simulink model "emldemo_bus_struct"  (Simulink 7.6)
settings: Solver=FixedStepDiscrete  StartTime=0.0  StopTime=1  FixedStep=1  RelTol=1e-3
PreLoadFcn:
  | load businfo.mat;
settings Model: Creator=The MathWorks Inc.
settings OptimizationCC: InitFltsAndDblsToZero=on
settings DebuggingCC: SaveWithParameterizedLinksMsg=none  SignalResolutionControl=TryResolveAllWithWarning  StrictBusMsg=Warning
settings SFSimCC: SimParseCustomCode=off
settings GRTTargetCC: TargetFcnLib=ansi_tfl_tmw.mat

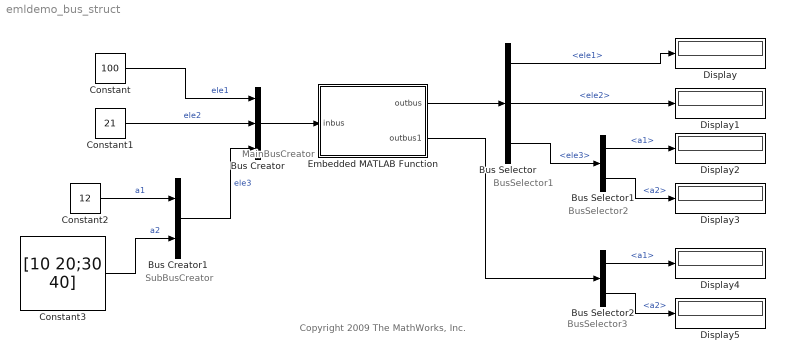
== system emldemo_bus_struct ==
  note: BusSelector1
  note: SubBusCreator
  note: MainBusCreator
  note: BusSelector2
  note: BusSelector3
  note: Copyright 2009 The MathWorks, Inc.
  Bus Creator : BusCreator  Inputs=3  OutDataTypeStr=Bus: MainBus  NonVirtualBus=on
  Bus Creator1 : BusCreator  Inputs=2  OutDataTypeStr=Bus: SubBus  NonVirtualBus=on
  Bus Selector : BusSelector  OutputSignals=ele1,ele2,ele3
  Bus Selector1 : BusSelector  OutputSignals=a1,a2
  Bus Selector2 : BusSelector  OutputSignals=a1,a2
  Constant : Constant  Value=100  OutDataTypeStr=double
  Constant1 : Constant  Value=21  OutDataTypeStr=single
  Constant2 : Constant  Value=12  OutDataTypeStr=double
  Constant3 : Constant  Value=[10 20;30 40]  OutDataTypeStr=int8
  Display{,1..5} (6 alike) : Display
  Embedded MATLAB Function : Stateflow chart  TreatAsAtomicUnit=on
  wires:
  Constant/1 -> Bus Creator/1  "ele1"
  Constant1/1 -> Bus Creator/2  "ele2"
  Bus Creator1/1 -> Bus Creator/3  "ele3"
  Constant2/1 -> Bus Creator1/1  "a1"
  Constant3/1 -> Bus Creator1/2  "a2"
  Bus Creator/1 -> Embedded MATLAB Function/1(inbus)
  Embedded MATLAB Function/1(outbus) -> Bus Selector/1
  Bus Selector/1 -> Display/1  "<ele1>"
  Bus Selector/2 -> Display1/1  "<ele2>"
  Bus Selector/3 -> Bus Selector1/1  "<ele3>"
  Bus Selector1/1 -> Display2/1  "<a1>"
  Bus Selector1/2 -> Display3/1  "<a2>"
  Bus Selector2/1 -> Display4/1  "<a1>"
  Bus Selector2/2 -> Display5/1  "<a2>"
  Embedded MATLAB Function/2(outbus1) -> Bus Selector2/1

== matlab function Embedded MATLAB Function ==
  data: inbus input double; outbus output Bus: MainBus size=1; outbus1 output Bus: SubBus size=1
function [outbus, outbus1] = fcn(inbus)
%#eml

substruct.a1 = inbus.ele3.a1;
substruct.a2 = int8([1 2;3 4]);

mystruct = struct('ele1',20.5, 'ele2', single(100), 'ele3', substruct);

outbus = mystruct;
outbus.ele3.a2 = 2*(substruct.a2);

outbus1 = inbus.ele3;
